simulink model "lab2"  (R2019a)
settings: Solver=FixedStepAuto  StartTime=0.0  StopTime=5  FixedStep=0.01  RelTol=1e-3
settings Model: Creator=Lenovo  LastModifiedBy=Lenovo

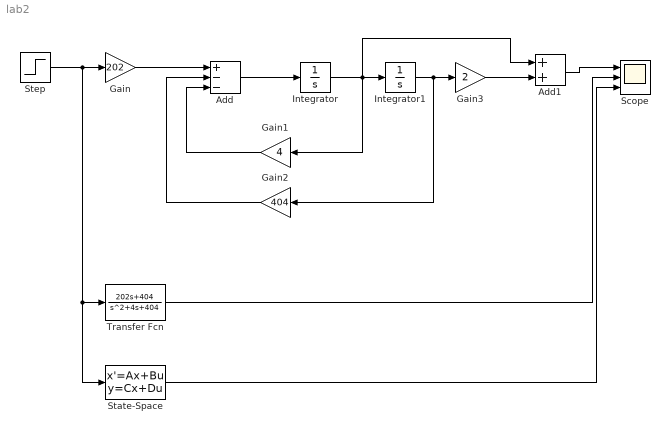
== system lab2 ==
  Add : Sum  Inputs=+--
  Add1 : Sum
  Gain : Gain  Gain=202
  Gain1 : Gain  Gain=4
  Gain2 : Gain  Gain=404
  Gain3 : Gain  Gain=2
  Integrator : Integrator
  Integrator1 : Integrator
  Scope : Scope  NumInputPorts=3
  State-Space : StateSpace  A=[0,1;-404,-4]  B=[0;202]  C=[2,1]  D=0  InitialCondition=0
  Step : Step  Time=0  SampleTime=0
  Transfer Fcn : TransferFcn  Numerator=[202, 404]  Denominator=[1 4 404]
  wires:
  Step/1 -> State-Space/1, Transfer Fcn/1, Gain/1
  Gain/1 -> Add/1
  Gain1/1 -> Add/3
  Gain2/1 -> Add/2
  Add/1 -> Integrator/1
  Gain3/1 -> Add1/2
  Integrator/1 -> Add1/1, Gain1/1, Integrator1/1
  Integrator1/1 -> Gain2/1, Gain3/1
  Add1/1 -> Scope/1
  Transfer Fcn/1 -> Scope/2
  State-Space/1 -> Scope/3
